simulink model "Simplified_Model_test"  (R2014a)
settings: Solver=ode45  StartTime=0.0  StopTime=10.0  RelTol=1e-3
libraries: simulink x3
settings Model: Creator=scorpii  LastModifiedBy=scorpii

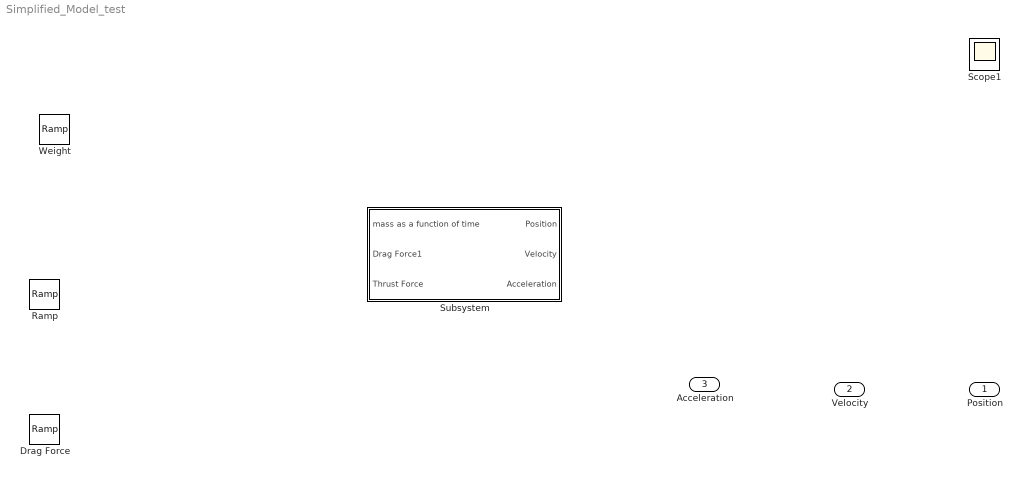
== system Simplified_Model_test ==
  Drag Force : simulink/Sources/Ramp  slope=0.5  start=0  X0=0
  Ramp : simulink/Sources/Ramp  slope=2  start=0  X0=0
  Scope1 : Scope
  Subsystem : Subsystem
  Weight : simulink/Sources/Ramp  slope=-1  start=0  X0=5
  Position : Outport
  Velocity : Outport  Port=2
  Acceleration : Outport  Port=3
  wires:
  ? -> ?

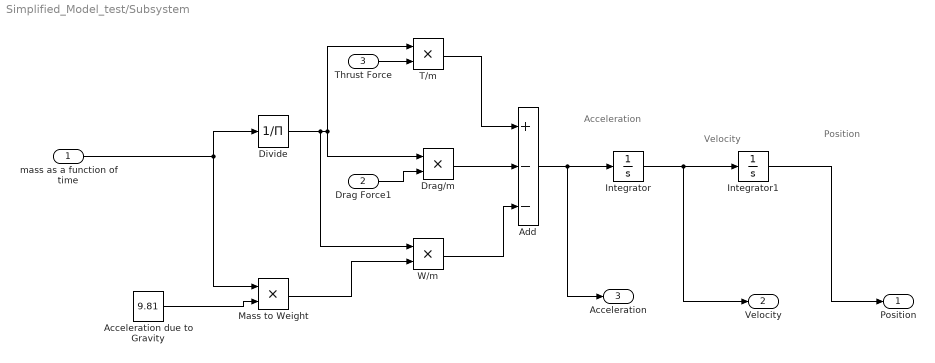
== system Simplified_Model_test/Subsystem ==
  note: Velocity
  note: Position
  note: Acceleration
  mass as a function of time : Inport
  Drag Force1 : Inport  Port=2
  Thrust Force : Inport  Port=3
  Acceleration due to Gravity : Constant  Value=9.81
  Add : Sum  Inputs=+--
  Divide : Product  Inputs=/
  Drag/m : Product
  Integrator : Integrator
  Integrator1 : Integrator
  Mass to Weight : Product
  T/m : Product
  W/m : Product
  Position : Outport
  Velocity : Outport  Port=2
  Acceleration : Outport  Port=3
  wires:
  W/m/1 -> Add/3
  T/m/1 -> Add/1
  Drag Force1/1 -> Drag/m/2
  Divide/1 -> Drag/m/1, T/m/1, W/m/1
  Integrator/1 -> Velocity/1, Integrator1/1
  mass as a function of time/1 -> Mass to Weight/1, Divide/1
  Integrator1/1 -> Position/1
  Thrust Force/1 -> T/m/2
  Add/1 -> Acceleration/1, Integrator/1
  Acceleration due to Gravity/1 -> Mass to Weight/2
  Drag/m/1 -> Add/2
  Mass to Weight/1 -> W/m/2
